simulink model "Assignment_1_full_system"  (R2023b)
settings: Solver=VariableStepAuto  StartTime=0.0  StopTime=320  RelTol=1e-3
libraries: simulink x5
settings Model: Creator=User  LastModifiedBy=User

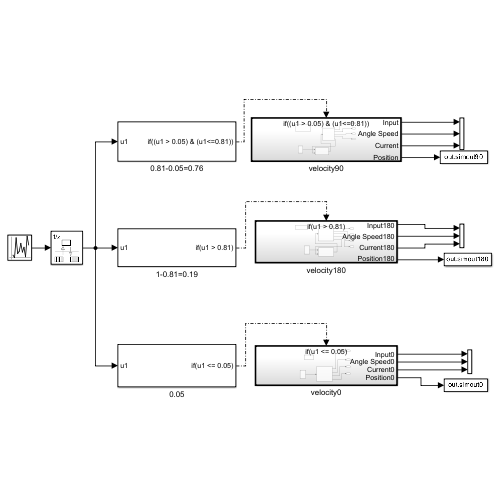
[thumbnail: Simulink's stored preview of the top-level diagram]
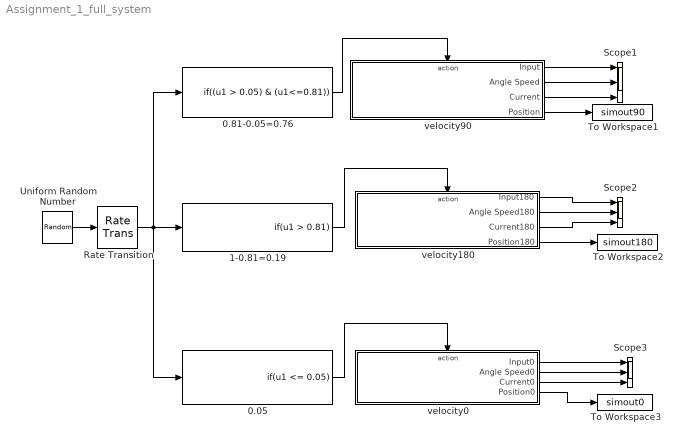
== system Assignment_1_full_system ==
  0.05 : If  IfExpression=u1 <= 0.05  ShowElse=off
  0.81-0.05=0.76 : If  IfExpression=(u1 > 0.05) & (u1<=0.81)  ShowElse=off
  1-0.81=0.19 : If  IfExpression=u1 > 0.81  ShowElse=off
  Rate Transition : RateTransition
  Scope1 : Scope  NumInputPorts=3
  Scope2 : Scope  NumInputPorts=3
  Scope3 : Scope  NumInputPorts=3
  To Workspace1 : ToWorkspace  VariableName=simout90  SaveFormat=Timeseries  SampleTime=-1
  To Workspace2 : ToWorkspace  VariableName=simout180  SaveFormat=Timeseries  SampleTime=-1
  To Workspace3 : ToWorkspace  VariableName=simout0  SaveFormat=Timeseries  SampleTime=-1
  Uniform Random Number : UniformRandomNumber  Minimum=0  Seed=16  SampleTime=16
  velocity0 : Subsystem  TreatAsAtomicUnit=on
  velocity180 : Subsystem  TreatAsAtomicUnit=on
  velocity90 : Subsystem  TreatAsAtomicUnit=on
  wires:
  Uniform Random Number/1 -> Rate Transition/1
  Rate Transition/1 -> 1-0.81=0.19/1, 0.81-0.05=0.76/1, 0.05/1
  velocity180/4(Position180) -> To Workspace2/1
  velocity180/2(Angle Speed180) -> Scope2/2
  velocity180/1(Input180) -> Scope2/1
  velocity180/3(Current180) -> Scope2/3
  1-0.81=0.19/1 -> velocity180/Action
  0.81-0.05=0.76/1 -> velocity90/Action
  velocity90/1(Input) -> Scope1/1
  velocity90/2(Angle Speed) -> Scope1/2
  velocity90/3(Current) -> Scope1/3
  velocity90/4(Position) -> To Workspace1/1
  0.05/1 -> velocity0/Action
  velocity0/1(Input0) -> Scope3/1
  velocity0/3(Current0) -> Scope3/3
  velocity0/2(Angle Speed0) -> Scope3/2
  velocity0/4(Position0) -> To Workspace3/1

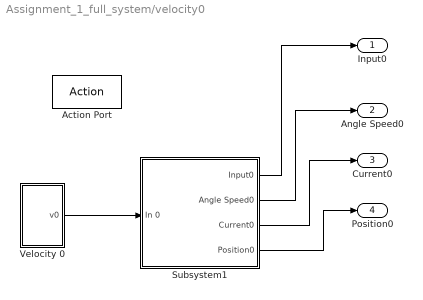
== system Assignment_1_full_system/velocity0 ==
  Action Port : ActionPort  ActionPortLabel=if(u1 <= 0.05)
  Subsystem1 : Subsystem
  Velocity 0 : Subsystem
  Input0 : Outport
  Angle Speed0 : Outport  Port=2
  Current0 : Outport  Port=3
  Position0 : Outport  Port=4
  wires:
  Subsystem1/1(Input0) -> Input0/1
  Subsystem1/3(Current0) -> Current0/1
  Subsystem1/2(Angle Speed0) -> Angle Speed0/1
  Subsystem1/4(Position0) -> Position0/1
  Velocity 0/1(v0) -> Subsystem1/1(In 0)

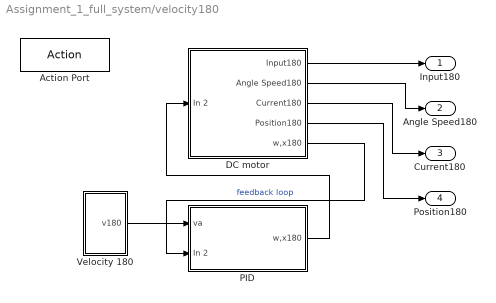
== system Assignment_1_full_system/velocity180 ==
  Action Port : ActionPort  ActionPortLabel=if(u1 > 0.81)
  DC motor : Subsystem
  PID : Subsystem
  Velocity 180 : Subsystem
  Input180 : Outport
  Angle Speed180 : Outport  Port=2
  Current180 : Outport  Port=3
  Position180 : Outport  Port=4
  wires:
  PID/1(w,x180) -> DC motor/1(In 2)
  DC motor/5(w,x180) -> PID/2(In 2)  "feedback loop"
  DC motor/4(Position180) -> Position180/1
  DC motor/2(Angle Speed180) -> Angle Speed180/1
  DC motor/3(Current180) -> Current180/1
  DC motor/1(Input180) -> Input180/1
  Velocity 180/1(v180) -> PID/1(va)

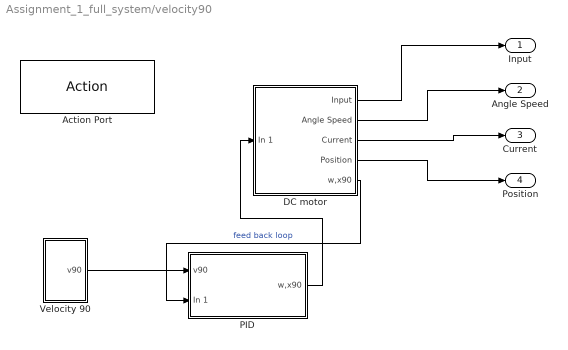
== system Assignment_1_full_system/velocity90 ==
  Action Port : ActionPort  ActionPortLabel=if((u1 > 0.05) & (u1<=0.81))
  DC motor : Subsystem
  PID : Subsystem
  Velocity 90 : Subsystem
  Input : Outport
  Angle Speed : Outport  Port=2
  Current : Outport  Port=3
  Position : Outport  Port=4
  wires:
  Velocity 90/1(v90) -> PID/1(v90)
  PID/1(w,x90) -> DC motor/1(In 1)
  DC motor/3(Current) -> Current/1
  DC motor/2(Angle Speed) -> Angle Speed/1
  DC motor/1(Input) -> Input/1
  DC motor/4(Position) -> Position/1
  DC motor/5(w,x90) -> PID/2(In 1)  "feed back loop"

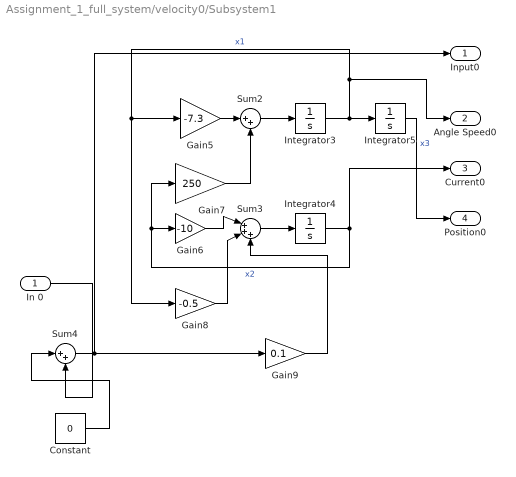
== system Assignment_1_full_system/velocity0/Subsystem1 ==
  In 0 : Inport
  Constant : Constant  Value=0
  Gain5 : Gain  Gain=-7.3
  Gain6 : Gain  Gain=-10
  Gain7 : Gain  Gain=250
  Gain8 : Gain  Gain=-0.5
  Gain9 : Gain  Gain=0.1
  Integrator3 : Integrator
  Integrator4 : Integrator
  Integrator5 : Integrator
  Sum2 : Sum  Inputs=|++
  Sum3 : Sum  Inputs=|+++
  Sum4 : Sum  Inputs=|++
  Input0 : Outport
  Angle Speed0 : Outport  Port=2
  Current0 : Outport  Port=3
  Position0 : Outport  Port=4
  wires:
  Integrator4/1 -> Current0/1, Gain7/1, Gain6/1  "x2"
  Gain7/1 -> Sum2/2
  Gain6/1 -> Sum3/1
  Sum2/1 -> Integrator3/1
  Gain9/1 -> Sum3/3
  Gain8/1 -> Sum3/2
  Sum3/1 -> Integrator4/1
  Integrator3/1 -> Angle Speed0/1, Gain8/1, Gain5/1, Integrator5/1  "x1"
  Gain5/1 -> Sum2/1
  Sum4/1 -> Input0/1, Gain9/1
  Constant/1 -> Sum4/1
  In 0/1 -> Sum4/2
  Integrator5/1 -> Position0/1  "x3"

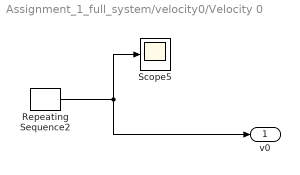
== system Assignment_1_full_system/velocity0/Velocity 0 ==
  Repeating Sequence2 : simulink/Sources/Repeating Sequence  rep_seq_t=[0 16]  rep_seq_y=[0 0]
  Scope5 : Scope
  v0 : Outport
  wires:
  Repeating Sequence2/1 -> v0/1, Scope5/1

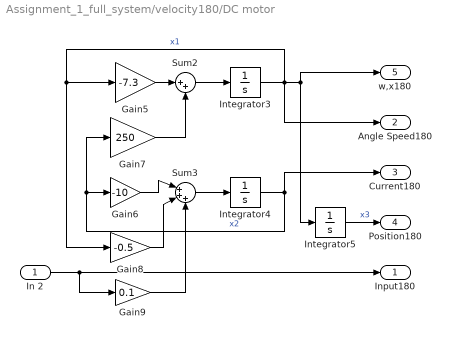
== system Assignment_1_full_system/velocity180/DC motor ==
  In 2 : Inport
  Gain5 : Gain  Gain=-7.3
  Gain6 : Gain  Gain=-10
  Gain7 : Gain  Gain=250
  Gain8 : Gain  Gain=-0.5
  Gain9 : Gain  Gain=0.1
  Integrator3 : Integrator
  Integrator4 : Integrator
  Integrator5 : Integrator
  Sum2 : Sum  Inputs=|++
  Sum3 : Sum  Inputs=|+++
  Input180 : Outport
  Angle Speed180 : Outport  Port=2
  Current180 : Outport  Port=3
  Position180 : Outport  Port=4
  w,x180 : Outport  Port=5
  wires:
  Integrator4/1 -> Current180/1, Gain7/1, Gain6/1  "x2"
  Gain7/1 -> Sum2/2
  Gain6/1 -> Sum3/1
  Sum2/1 -> Integrator3/1
  Gain9/1 -> Sum3/3
  Gain8/1 -> Sum3/2
  Sum3/1 -> Integrator4/1
  Integrator3/1 -> Gain8/1, Gain5/1, Angle Speed180/1, Integrator5/1, w,x180/1  "x1"
  Gain5/1 -> Sum2/1
  Integrator5/1 -> Position180/1  "x3"
  In 2/1 -> Gain9/1, Input180/1

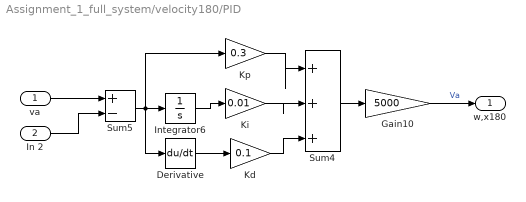
== system Assignment_1_full_system/velocity180/PID ==
  va : Inport
  In 2 : Inport  Port=2
  Derivative : Derivative
  Gain10 : Gain  Gain=5000
  Integrator6 : Integrator
  Kd : Gain  Gain=0.1
  Ki : Gain  Gain=0.01
  Kp : Gain  Gain=0.3
  Sum4 : Sum  Inputs=|+++
  Sum5 : Sum  Inputs=+-
  w,x180 : Outport
  wires:
  Kp/1 -> Sum4/1
  Derivative/1 -> Kd/1
  Sum5/1 -> Integrator6/1, Kp/1, Derivative/1
  Ki/1 -> Sum4/2
  va/1 -> Sum5/1
  Sum4/1 -> Gain10/1
  Gain10/1 -> w,x180/1  "Va"
  Kd/1 -> Sum4/3
  Integrator6/1 -> Ki/1
  In 2/1 -> Sum5/2

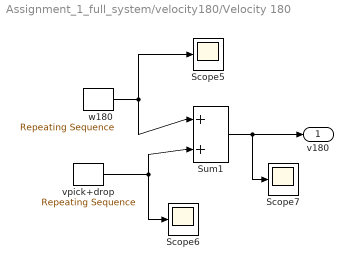
== system Assignment_1_full_system/velocity180/Velocity 180 ==
  Scope5 : Scope
  Scope6 : Scope
  Scope7 : Scope
  Sum1 : Sum  Inputs=|++
  vpick+drop : simulink/Sources/Repeating Sequence  rep_seq_t=[0 0.25 1 1.25 1.5 1.75 2.5 2.75 3 16]  rep_seq_y=[0 pi/2 pi/2 0 0 -pi/2 -pi/2 0 0 0]
  w180 : simulink/Sources/Repeating Sequence  rep_seq_t="[0 3 3.25 5  5.25 5.5 5.75 7.5 7.75 8 16]"  rep_seq_y=[0 0 pi/2 pi/2 0 0 -pi/2 -pi/2 0 0 0]
  v180 : Outport
  wires:
  w180/1 -> Sum1/1, Scope5/1
  Sum1/1 -> v180/1, Scope7/1
  vpick+drop/1 -> Scope6/1, Sum1/2

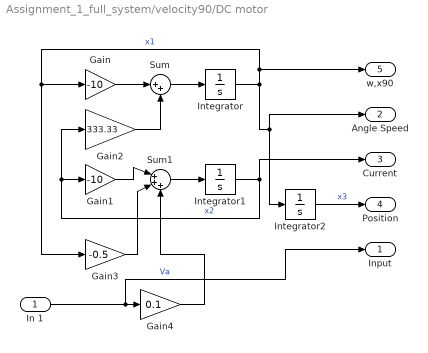
== system Assignment_1_full_system/velocity90/DC motor ==
  In 1 : Inport
  Gain : Gain  Gain=-10
  Gain1 : Gain  Gain=-10
  Gain2 : Gain  Gain=333.33
  Gain3 : Gain  Gain=-0.5
  Gain4 : Gain  Gain=0.1
  Integrator : Integrator
  Integrator1 : Integrator
  Integrator2 : Integrator
  Sum : Sum  Inputs=|++
  Sum1 : Sum  Inputs=|+++
  Input : Outport
  Angle Speed : Outport  Port=2
  Current : Outport  Port=3
  Position : Outport  Port=4
  w,x90 : Outport  Port=5
  wires:
  Integrator/1 -> Gain/1, Gain3/1, w,x90/1, Angle Speed/1, Integrator2/1  "x1"
  Sum1/1 -> Integrator1/1
  Gain/1 -> Sum/1
  Sum/1 -> Integrator/1
  Gain4/1 -> Sum1/3
  Integrator1/1 -> Current/1, Gain2/1, Gain1/1  "x2"
  Gain3/1 -> Sum1/2
  Integrator2/1 -> Position/1  "x3"
  Gain1/1 -> Sum1/1
  Gain2/1 -> Sum/2
  In 1/1 -> Input/1, Gain4/1  "Va"

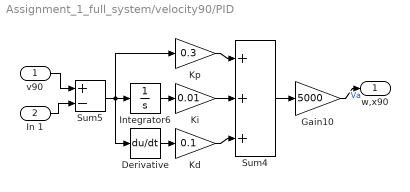
== system Assignment_1_full_system/velocity90/PID ==
  v90 : Inport
  In 1 : Inport  Port=2
  Derivative : Derivative
  Gain10 : Gain  Gain=5000
  Integrator6 : Integrator
  Kd : Gain  Gain=0.1
  Ki : Gain  Gain=0.01
  Kp : Gain  Gain=0.3
  Sum4 : Sum  Inputs=|+++
  Sum5 : Sum  Inputs=+-
  w,x90 : Outport
  wires:
  Kp/1 -> Sum4/1
  Derivative/1 -> Kd/1
  Sum5/1 -> Kp/1, Integrator6/1, Derivative/1
  Ki/1 -> Sum4/2
  Sum4/1 -> Gain10/1
  Gain10/1 -> w,x90/1  "Va"
  Kd/1 -> Sum4/3
  Integrator6/1 -> Ki/1
  In 1/1 -> Sum5/2
  v90/1 -> Sum5/1

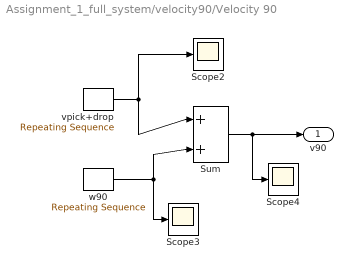
== system Assignment_1_full_system/velocity90/Velocity 90 ==
  Scope2 : Scope
  Scope3 : Scope
  Scope4 : Scope
  Sum : Sum  Inputs=|++
  vpick+drop : simulink/Sources/Repeating Sequence  rep_seq_t=[0 0.25 1 1.25 1.5 1.75 2.5 2.75 3 16]  rep_seq_y=[0 pi/2 pi/2 0 0 -pi/2 -pi/2 0 0 0]
  w90 : simulink/Sources/Repeating Sequence  rep_seq_t=[0 3 3.25 4 4.25 4.5 4.75 5.5 5.75 6 16]  rep_seq_y=[0 0 pi/2 pi/2 0 0 -pi/2 -pi/2 0 0 0]
  v90 : Outport
  wires:
  vpick+drop/1 -> Sum/1, Scope2/1
  w90/1 -> Sum/2, Scope3/1
  Sum/1 -> v90/1, Scope4/1
